simulink model "Test"  (R2020b)
settings: Solver=VariableStepAuto  StartTime=0.0  StopTime=10.0  RelTol=1e-3
undefined symbols (not defined in the file or in its folder): smiData, X, Y, Z
libraries: sm_lib x109, nesl_utility x16, simulink_extras x8
(part 3 of 3)

== matlab function Test/ Dynamics ==
  data: pos input; tau output; vel input; acc input
function tau = tauFunction(pos, vel, acc)

theta1 = pos(1)*pi/180; 
theta2 = pos(2)*pi/180;
theta3 = pos(3)*pi/180; 
theta4 = pos(4)*pi/180;

d_theta1 = vel(1); 
d_theta2 = vel(2); 
d_theta3 = vel(3); 
d_theta4 = vel(4);

dd_theta1 = acc(1); 
dd_theta2 = acc(2); 
dd_theta3 = acc(3); 
dd_theta4 = acc(4); 

EOMFinal = [0.0000089496200000000012287487693996013*d_theta2^2*sin(theta2) - dd_theta1*(0.0027559110003139361176579076962264*cos(2.0*theta2 + theta3 + theta4 - 0.37778562010271929275313377711607) - 0.0027559110003139361176579076962264*cos(theta3 + theta4 - 0.37778562010271929275313377711607) + 0.012009011246003126444392396437535*cos(2.0*theta2 - 0.0017368216299427074441940157622878) + 0.0083738512*cos(2.0*theta2 + theta3) + 0.0026429543340982030361376297942926*cos(2.0*theta2 + 2.0*theta3 + 0.0017692823441303055913378980616204) + 0.0004873367282*cos(2.0*theta2 + 2.0*theta3 + 2.0*theta4 - 0.75557124020543858550626755423214) - 0.0018414496229370391331623292333876*cos(theta4 - 0.37778562010271929275313377711607) + 0.0018414496229370391331623292333876*cos(2.0*theta2 + 2.0*theta3 + theta4 - 0.37778562010271929275313377711607) - 0.0083738512*cos(theta3) - 0.015436564708719999986146902997142) - 7.1746481373430634031294954664444e-43*dd_theta1*cos(2*theta2 + 2*theta3) - 1.7936620343357658507823738666111e-43*dd_theta1*sin(2.0*theta2 + 2.0*theta3 + theta4) + 1.4012984643248170709237295832899e-45*dd_theta1*sin(2*theta2 + 2*theta3) - dd_theta2*(0.00000022549466202107757928824911443453*cos(theta2 + theta3 + 0.006430351742384142739604312207095) + 0.0000089502182238647132325573496145577*cos(theta2 + 0.011561986867147647360931077407364)) - dd_theta3*(0.00000022549466202107757928824911443453*cos(theta2 + theta3 + 0.006430351742384142739604312207095) + 0.0000044751091119323566162786748072789*cos(theta2 + 0.011561986867147647360931077407364)) - 0.0000044751091119323566162786748072789*dd_theta4*cos(theta2 + 0.011561986867147647360931077407364) - 4.379057701015053346636654947781e-47*dd_theta2*cos(theta2 + theta3) + 7.1746481373430634031294954664444e-43*dd_theta1*cos(theta3 + theta4) - 4.379057701015053346636654947781e-47*dd_theta3*cos(theta2 + theta3) - 7.1746481373430634031294954664444e-43*dd_theta1*cos(2.0*theta2 + theta3 + theta4) + 2.8025969286496341418474591665798e-45*dd_theta2*cos(theta2) + 1.4012984643248170709237295832899e-45*dd_theta3*cos(theta2) + 1.4012984643248170709237295832899e-45*dd_theta4*cos(theta2) + 1.7936620343357658507823738666111e-43*dd_theta1*sin(theta4) + 0.0000000014499999999999999558914580739138*d_theta2^2*cos(theta2 + theta3) + 0.0000000014499999999999999558914580739138*d_theta3^2*cos(theta2 + theta3) + 0.00000022549000000000001604358518866172*d_theta2^2*sin(theta2 + theta3) + 0.00000022549000000000001604358518866172*d_theta3^2*sin(theta2 + theta3) + 0.00000010347999999999999751962027460389*d_theta2^2*cos(theta2) + 0.000000051739999999999998759810137301946*d_theta2*d_theta3*cos(theta2) + 0.000000051739999999999998759810137301946*d_theta2*d_theta4*cos(theta2) + 0.0006792429*d_theta1*d_theta4*cos(theta4) - 0.0083738512*d_theta1*d_theta3*sin(theta3) + 0.0000044748100000000006143743846998007*d_theta2*d_theta3*sin(theta2) + 0.0000044748100000000006143743846998007*d_theta2*d_theta4*sin(theta2) - 0.00171159744*d_theta1*d_theta4*sin(theta4) - 0.000668338048*d_theta1*d_theta2*cos(2*theta2 + 2*theta3 + 2*theta4) - 0.000668338048*d_theta1*d_theta3*cos(2*theta2 + 2*theta3 + 2*theta4) - 0.000668338048*d_theta1*d_theta4*cos(2*theta2 + 2*theta3 + 2*theta4) + 0.0007094452764*d_theta1*d_theta2*sin(2*theta2 + 2*theta3 + 2*theta4) + 0.0007094452764*d_theta1*d_theta3*sin(2*theta2 + 2*theta3 + 2*theta4) + 0.0007094452764*d_theta1*d_theta4*sin(2*theta2 + 2*theta3 + 2*theta4) + 0.0167477024*d_theta1*d_theta2*sin(2.0*theta2 + theta3) + 0.0083738512*d_theta1*d_theta3*sin(2.0*theta2 + theta3) - 0.0013584858*d_theta1*d_theta2*cos(2.0*theta2 + 2.0*theta3 + theta4) - 0.0013584858*d_theta1*d_theta3*cos(2.0*theta2 + 2.0*theta3 + theta4) - 0.0006792429*d_theta1*d_theta4*cos(2.0*theta2 + 2.0*theta3 + theta4) + 0.0000093522600000000008160653056088485*d_theta1*d_theta2*cos(2*theta2 + 2*theta3) + 0.0000093522600000000008160653056088485*d_theta1*d_theta3*cos(2*theta2 + 2*theta3) + 0.00342319488*d_theta1*d_theta2*sin(2.0*theta2 + 2.0*theta3 + theta4) + 0.00342319488*d_theta1*d_theta3*sin(2.0*theta2 + 2.0*theta3 + theta4) + 0.00171159744*d_theta1*d_theta4*sin(2.0*theta2 + 2.0*theta3 + theta4) - 0.000041715000000000002945699240086697*d_theta1*d_theta2*cos(2.0*theta2) + 0.005285900394799999988342437307054*d_theta1*d_theta2*sin(2*theta2 + 2*theta3) + 0.005285900394799999988342437307054*d_theta1*d_theta3*sin(2*theta2 + 2*theta3) + 0.024017986266239999957260424787719*d_theta1*d_theta2*sin(2.0*theta2) + 0.0000000028999999999999999117829161478276*d_theta2*d_theta3*cos(theta2 + theta3) + 0.001016554*d_theta1*d_theta3*cos(theta3 + theta4) + 0.001016554*d_theta1*d_theta4*cos(theta3 + theta4) + 0.00000045098000000000003208717037732345*d_theta2*d_theta3*sin(theta2 + theta3) - 0.0025615744*d_theta1*d_theta3*sin(theta3 + theta4) - 0.0025615744*d_theta1*d_theta4*sin(theta3 + theta4) - 0.002033108*d_theta1*d_theta2*cos(2.0*theta2 + theta3 + theta4) - 0.001016554*d_theta1*d_theta3*cos(2.0*theta2 + theta3 + theta4) - 0.001016554*d_theta1*d_theta4*cos(2.0*theta2 + theta3 + theta4) + 0.0051231488*d_theta1*d_theta2*sin(2.0*theta2 + theta3 + theta4) + 0.0025615744*d_theta1*d_theta3*sin(2.0*theta2 + theta3 + theta4) + 0.0025615744*d_theta1*d_theta4*sin(2.0*theta2 + theta3 + theta4)
                                                                                                                                                                                                                                                                                                                                                                                                                                                                                                                                                                                                                                                                                                                                                                                                                                                                                                                                                                                                                                                                                                                                                                                                                                                                                                                                                                                                                                                                                                                                                                                                                                                                                                                                                               0.12301384555946751216091206171338*cos(theta2 + theta3 + theta4 + 1.1930107066921773264781879145237) - 0.3737782672*sin(theta2 + theta3) - 1.07697499416*sin(theta2) - 0.0083738512*d_theta3^2*sin(theta3) - 0.00171159744*d_theta4^2*sin(theta4) + dd_theta3*(0.0027559110003139361176579076962264*cos(theta3 + theta4 - 0.37778562010271929275313377711607) + 0.0036828992458740782663246584667753*cos(theta4 - 0.37778562010271929275313377711607) + 0.0083738512*cos(theta3) + 0.0063988872611999999919430743178239) + dd_theta2*(0.0055118220006278722353158153924528*cos(theta3 + theta4 - 0.37778562010271929275313377711607) + 0.0036828992458740782663246584667753*cos(theta4 - 0.37778562010271929275313377711607) + 0.0167477024*cos(theta3) + 0.028215028667439999995747989034456) - dd_theta1*(0.00000022549466202107757928824911443453*cos(theta2 + theta3 + 0.006430351742384142739604312207095) + 0.0000089502182238647132325573496145577*cos(theta2 + 0.011561986867147647360931077407364)) + 0.000334169024*d_theta1^2*cos(2*theta2 + 2*theta3 + 2*theta4) - 4.379057701015053346636654947781e-47*dd_theta1*cos(theta2 + theta3) + 1.4349296274686126806258990932889e-42*dd_theta2*cos(theta3 + theta4) + 7.1746481373430634031294954664444e-43*dd_theta3*cos(theta3 + theta4) + 7.1746481373430634031294954664444e-43*dd_theta4*cos(theta3 + theta4) - 0.0003547226382*d_theta1^2*sin(2*theta2 + 2*theta3 + 2*theta4) - 0.0083738512*d_theta1^2*sin(2.0*theta2 + theta3) + 0.0006792429*d_theta1^2*cos(2.0*theta2 + 2.0*theta3 + theta4) - 0.0000046761300000000004080326528044242*d_theta1^2*cos(2*theta2 + 2*theta3) - 0.00171159744*d_theta1^2*sin(2.0*theta2 + 2.0*theta3 + theta4) + 0.000020857500000000001472849620043348*d_theta1^2*cos(2.0*theta2) + 2.8025969286496341418474591665798e-45*dd_theta1*cos(theta2) - 0.002642950197399999994171218653527*d_theta1^2*sin(2*theta2 + 2*theta3) + dd_theta4*(0.0027559110003139361176579076962264*cos(theta3 + theta4 - 0.37778562010271929275313377711607) + 0.0018414496229370391331623292333876*cos(theta4 - 0.37778562010271929275313377711607) + 0.0010940804564000000038049147166319) - 0.01200899313311999997863021239386*d_theta1^2*sin(2.0*theta2) + 3.5873240686715317015647477332222e-43*dd_theta2*sin(theta4) + 3.5873240686715317015647477332222e-43*dd_theta3*sin(theta4) + 1.7936620343357658507823738666111e-43*dd_theta4*sin(theta4) + 0.001016554*d_theta3^2*cos(theta3 + theta4) + 0.001016554*d_theta4^2*cos(theta3 + theta4) - 0.0025615744*d_theta3^2*sin(theta3 + theta4) - 0.0025615744*d_theta4^2*sin(theta3 + theta4) + 0.001016554*d_theta1^2*cos(2.0*theta2 + theta3 + theta4) - 0.0025615744*d_theta1^2*sin(2.0*theta2 + theta3 + theta4) + 0.0006792429*d_theta4^2*cos(theta4) - 0.000000051739999999999998759810137301946*d_theta1*d_theta3*cos(theta2) - 0.000000051739999999999998759810137301946*d_theta1*d_theta4*cos(theta2) + 0.0013584858*d_theta2*d_theta4*cos(theta4) + 0.0013584858*d_theta3*d_theta4*cos(theta4) - 0.0000044748100000000006143743846998007*d_theta1*d_theta3*sin(theta2) - 0.0000044748100000000006143743846998007*d_theta1*d_theta4*sin(theta2) - 0.0167477024*d_theta2*d_theta3*sin(theta3) - 0.00342319488*d_theta2*d_theta4*sin(theta4) - 0.00342319488*d_theta3*d_theta4*sin(theta4) + 0.002033108*d_theta2*d_theta3*cos(theta3 + theta4) + 0.002033108*d_theta2*d_theta4*cos(theta3 + theta4) + 0.002033108*d_theta3*d_theta4*cos(theta3 + theta4) - 0.0051231488*d_theta2*d_theta3*sin(theta3 + theta4) - 0.0051231488*d_theta2*d_theta4*sin(theta3 + theta4) - 0.0051231488*d_theta3*d_theta4*sin(theta3 + theta4)
                                                                                                                                                                                                                                                                                                                                                                                                                                                                                                                                                                                                                                                                                                                                                                                                                                                                                                                                                                                                                                                                                                                                                                                                                                                                                                                                                                                                                                                                                                                                                                                                                                                                                                                                                                                                                                                                                                                                                                                                                                                                                                                                                                                                                                                                                                                                                                                                                                                                                                                                                                                                                                                                                                                                                                                                   0.12301384555946751216091206171338*cos(theta2 + theta3 + theta4 + 1.1930107066921773264781879145237) - 0.3737782672*sin(theta2 + theta3) + 0.0041869256*d_theta1^2*sin(theta3) + 0.0083738512*d_theta2^2*sin(theta3) - 0.00171159744*d_theta4^2*sin(theta4) + dd_theta2*(0.0027559110003139361176579076962264*cos(theta3 + theta4 - 0.37778562010271929275313377711607) + 0.0036828992458740782663246584667753*cos(theta4 - 0.37778562010271929275313377711607) + 0.0083738512*cos(theta3) + 0.0063988872611999999919430743178239) - dd_theta1*(0.00000022549466202107757928824911443453*cos(theta2 + theta3 + 0.006430351742384142739604312207095) + 0.0000044751091119323566162786748072789*cos(theta2 + 0.011561986867147647360931077407364)) + 0.000334169024*d_theta1^2*cos(2*theta2 + 2*theta3 + 2*theta4) - 4.379057701015053346636654947781e-47*dd_theta1*cos(theta2 + theta3) + 7.1746481373430634031294954664444e-43*dd_theta2*cos(theta3 + theta4) - 0.0003547226382*d_theta1^2*sin(2*theta2 + 2*theta3 + 2*theta4) - 0.0041869256*d_theta1^2*sin(2.0*theta2 + theta3) + 0.0006792429*d_theta1^2*cos(2.0*theta2 + 2.0*theta3 + theta4) - 0.0000046761300000000004080326528044242*d_theta1^2*cos(2*theta2 + 2*theta3) - 0.00171159744*d_theta1^2*sin(2.0*theta2 + 2.0*theta3 + theta4) + 1.4012984643248170709237295832899e-45*dd_theta1*cos(theta2) - 0.002642950197399999994171218653527*d_theta1^2*sin(2*theta2 + 2*theta3) + 3.5873240686715317015647477332222e-43*dd_theta2*sin(theta4) + 3.5873240686715317015647477332222e-43*dd_theta3*sin(theta4) + 1.7936620343357658507823738666111e-43*dd_theta4*sin(theta4) - 0.000508277*d_theta1^2*cos(theta3 + theta4) - 0.001016554*d_theta2^2*cos(theta3 + theta4) + dd_theta4*(0.0018414496229370391331623292333876*cos(theta4 - 0.37778562010271929275313377711607) + 0.0010940804564000000038049147166319) + 0.0012807872*d_theta1^2*sin(theta3 + theta4) + 0.0025615744*d_theta2^2*sin(theta3 + theta4) + 0.000508277*d_theta1^2*cos(2.0*theta2 + theta3 + theta4) - 0.0012807872*d_theta1^2*sin(2.0*theta2 + theta3 + theta4) + 0.0006792429*d_theta4^2*cos(theta4) + dd_theta3*(0.0036828992458740782663246584667753*cos(theta4 - 0.37778562010271929275313377711607) + 0.0063988872611999999919430743178239) + 0.000000051739999999999998759810137301946*d_theta1*d_theta2*cos(theta2) + 0.0013584858*d_theta2*d_theta4*cos(theta4) + 0.0013584858*d_theta3*d_theta4*cos(theta4) + 0.0000044748100000000006143743846998007*d_theta1*d_theta2*sin(theta2) - 0.00342319488*d_theta2*d_theta4*sin(theta4) - 0.00342319488*d_theta3*d_theta4*sin(theta4)
                                                                                                                                                                                                                                                                                                                                                                                                                                                                                                                                                                                                                                                                                                                                                                                                                                                                                                                                                                                                                                                                                                                                                                                                                                                                                                                                                                                                                                                                                                                                                                                                                                                                                                                                                                                                                                                                                                                                                                                                                                                                                                                                                                                                                                                                                                                                                                                                                                                                                                                                                                                                                                                                                                                                                                                                                                                                                                                                                                                                                                                                                                                                                                                                                                                                                                                                                                                                                              0.0010940804564000000038049147166319*dd_theta4 + 0.12301384555946751216091206171338*cos(theta2 + theta3 + theta4 + 1.1930107066921773264781879145237) + 0.00085579872*d_theta1^2*sin(theta4) + 0.00171159744*d_theta2^2*sin(theta4) + 0.00171159744*d_theta3^2*sin(theta4) - 0.0000044751091119323566162786748072789*dd_theta1*cos(theta2 + 0.011561986867147647360931077407364) + 0.000334169024*d_theta1^2*cos(2*theta2 + 2*theta3 + 2*theta4) + 7.1746481373430634031294954664444e-43*dd_theta2*cos(theta3 + theta4) - 0.0003547226382*d_theta1^2*sin(2*theta2 + 2*theta3 + 2*theta4) + 0.00033962145*d_theta1^2*cos(2.0*theta2 + 2.0*theta3 + theta4) - 0.00085579872*d_theta1^2*sin(2.0*theta2 + 2.0*theta3 + theta4) + 1.4012984643248170709237295832899e-45*dd_theta1*cos(theta2) + dd_theta2*(0.0027559110003139361176579076962264*cos(theta3 + theta4 - 0.37778562010271929275313377711607) + 0.0018414496229370391331623292333876*cos(theta4 - 0.37778562010271929275313377711607) + 0.0010940804564000000038049147166319) + 1.7936620343357658507823738666111e-43*dd_theta2*sin(theta4) + 1.7936620343357658507823738666111e-43*dd_theta3*sin(theta4) - 0.000508277*d_theta1^2*cos(theta3 + theta4) - 0.001016554*d_theta2^2*cos(theta3 + theta4) + dd_theta3*(0.0018414496229370391331623292333876*cos(theta4 - 0.37778562010271929275313377711607) + 0.0010940804564000000038049147166319) + 0.0012807872*d_theta1^2*sin(theta3 + theta4) + 0.0025615744*d_theta2^2*sin(theta3 + theta4) + 0.000508277*d_theta1^2*cos(2.0*theta2 + theta3 + theta4) - 0.0012807872*d_theta1^2*sin(2.0*theta2 + theta3 + theta4) - 0.00033962145*d_theta1^2*cos(theta4) - 0.0006792429*d_theta2^2*cos(theta4) - 0.0006792429*d_theta3^2*cos(theta4) + 0.000000051739999999999998759810137301946*d_theta1*d_theta2*cos(theta2) - 0.0013584858*d_theta2*d_theta3*cos(theta4) + 0.0000044748100000000006143743846998007*d_theta1*d_theta2*sin(theta2) + 0.00342319488*d_theta2*d_theta3*sin(theta4)];
tau = [EOMFinal(1); EOMFinal(2); EOMFinal(3); EOMFinal(4)]

== matlab function Test/MATLAB Function3 ==
  data: t1 input; Pos output; t2 input; t3 input; t4 input
%% Crustecrwler forward kinematics
function Pos  = ForwardKinFunction(t1, t2, t3, t4)
theta1 = t1*pi/180;
theta2 = t2*pi/180;
theta3 = t3*pi/180;
theta4 = t4*pi/180;
% Denne section udregner Matricen T04, med de vinkler vi selv s?tter ind
% t1, t2, t3 og t4 beskriver theta vinklerne i hver motor
%Vinklerne inds?ttes i denavit hartenberg parameterne for vores robot:
T01=TDH(0,0,0,theta1+90*pi/180)
T12=TDH(-90*pi/180,0,0,theta2-90*pi/180)
T23=TDH(0,220,0,theta3);
T34=TDH(0,147,0,theta4);
%Base to final joint
T04=T01*T12*T23*T34;
Pos=[T04(1,4); T04(2,4); T04(3,4)]
